simulink model "sisfreqlinear"  (R2023b)
settings: Solver=VariableStepAuto  StartTime=0.0  StopTime=10.0  RelTol=1e-3
settings Model: Creator=Geovanne  LastModifiedBy=Geovanne

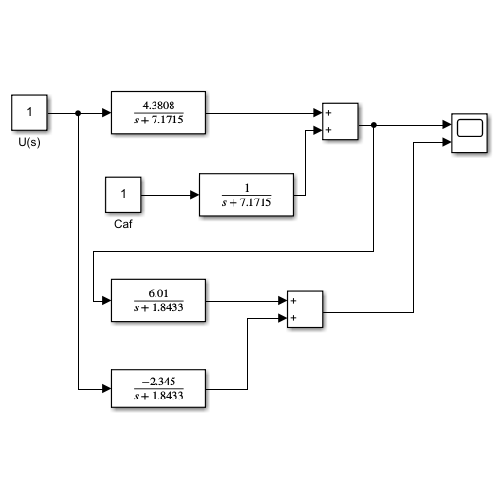
[thumbnail: Simulink's stored preview of the top-level diagram]
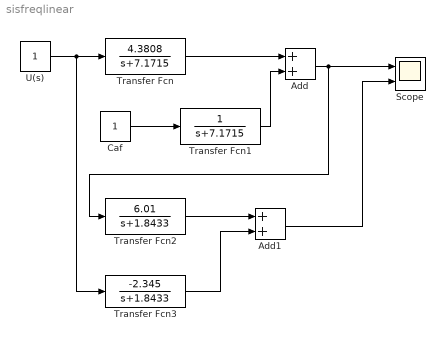
== system sisfreqlinear ==
  Add : Sum
  Add1 : Sum
  Caf : Constant
  Scope : Scope  NumInputPorts=2
  Transfer Fcn : TransferFcn  Numerator=[4.3808]  Denominator=[1 7.1715]
  Transfer Fcn1 : TransferFcn  Denominator=[1 7.1715]
  Transfer Fcn2 : TransferFcn  Numerator=[6.01]  Denominator=[1 1.8433]
  Transfer Fcn3 : TransferFcn  Numerator=[-2.345]  Denominator=[1 1.8433]
  U(s) : Constant
  wires:
  Transfer Fcn/1 -> Add/1
  U(s)/1 -> Transfer Fcn3/1, Transfer Fcn/1
  Transfer Fcn2/1 -> Add1/1
  Transfer Fcn3/1 -> Add1/2
  Transfer Fcn1/1 -> Add/2
  Add/1 -> Transfer Fcn2/1, Scope/1
  Add1/1 -> Scope/2
  Caf/1 -> Transfer Fcn1/1
